simulink model "BLDC_motor_control_v1"  (R2017b)
settings: Solver=FixedStepDiscrete  StartTime=0.0  StopTime=10  FixedStep=1e-5  RelTol=1e-3
values from neighbouring files (symbols this model uses):
  p = 2    [BLDC_model_init.m]
libraries: nesl_utility x41, fl_lib x33, pe_lib x30, simulink x6, pePwmGenerator x2
(part 1 of 2)
settings Model: SimulationMode=accelerator  Creator=proso  LastModifiedBy=proso

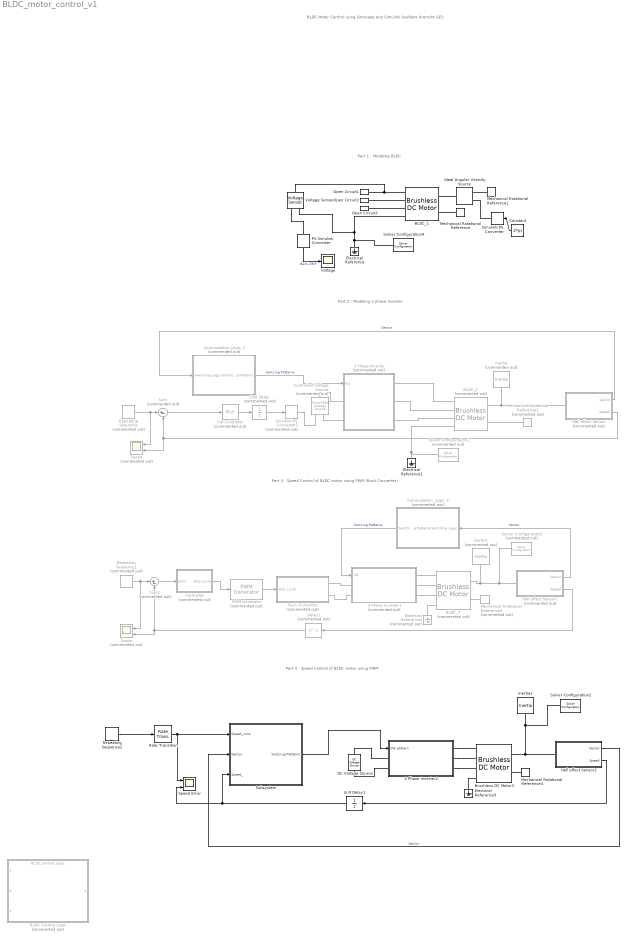
== system BLDC_motor_control_v1 ==
  note: BLDC Motor Control using Simscape and Simulink
      |
      | Soufiane Kremcht GE2
  note: Part 1 : Modeling BLDC
  note: Part 2 : Modeling 3 phase Inverter
  note: Part 3 : Speed Control of BLDC motor using PWM
      | (Buck Converter)
  note: Part 4 : Speed Control of BLDC motor using PWM
  3 Phase Inverter : Subsystem  Commented=on
  3 Phase Inverter1 : Subsystem  Commented=on
  3 Phase Inverter2 : Subsystem
  BLDC Control Logic : ModelReference  Commented=on  ModelNameDialog=BLDC_Control_Logic  SimulationMode=Normal  ModelReferenceVersion=1.23
  BLDC_1 : pe_lib/Machines/Permanent Magnet Rotor/Brushless DC Motor  rotor_param=1  pm_flux_linkage=1 Wb  theta_constant=120 deg  emf_max=9.6 V  DphiDtheta_tab=[0, -.1528, -.1528, .1528, .1528, 0] Wb/rad  back_emf_tab=[0, -9.6, -9.6, 9.6, 9.6, 0] V  rotor_angle_tab=[0, 7.5, 22.5, 37.5, 52.5, 60] deg  w_meas=600 rpm  nPolePairs=1  stator_param=1  Ld=8.5e-3 H  Lq=8.5e-3 H  L0=0 H  Ls=0.0002 H  Lm=0 H  Ms=0.00002 H  Rs=0.04 Ohm  initial_currents=[0, 0, 0] A  axes_param=2  angular_position0=0 deg
      settings: SourceProductName=Simscape Power Systems  SourceProductBaseCode=PS
  BLDC_2 : pe_lib/Machines/Permanent Magnet Rotor/Brushless DC Motor  Commented=on  rotor_param=1  pm_flux_linkage=1 Wb  theta_constant=60 deg  emf_max=9.6 V  DphiDtheta_tab=[0, -.1528, -.1528, .1528, .1528, 0] Wb/rad  back_emf_tab=[0, -9.6, -9.6, 9.6, 9.6, 0] V  rotor_angle_tab=[0, 7.5, 22.5, 37.5, 52.5, 60] deg  w_meas=600 rpm  nPolePairs=2  stator_param=1  Ld=8.5e-3 H  Lq=8.5e-3 H  L0=0 H  Ls=0.0002 H  Lm=0 H  Ms=0.00002 H  Rs=0.04 Ohm  initial_currents=[0, 0, 0] A  axes_param=2  angular_position0=0 deg
      settings: SourceProductName=Simscape Power Systems  SourceProductBaseCode=PS
  "BLDC_3 " : pe_lib/Machines/Permanent Magnet Rotor/Brushless DC Motor  Commented=on  rotor_param=1  pm_flux_linkage=1 Wb  theta_constant=120 deg  emf_max=9.6 V  DphiDtheta_tab=[0, -.1528, -.1528, .1528, .1528, 0] Wb/rad  back_emf_tab=[0, -9.6, -9.6, 9.6, 9.6, 0] V  rotor_angle_tab=[0, 7.5, 22.5, 37.5, 52.5, 60] deg  w_meas=600 rpm  nPolePairs=1  stator_param=1  Ld=8.5e-3 H  Lq=8.5e-3 H  L0=0 H  Ls=0.0002 H  Lm=0 H  Ms=0.00002 H  Rs=0.04 Ohm  initial_currents=[0, 0, 0] A  axes_param=2  angular_position0=0 deg
      settings: SourceProductName=Simscape Power Systems  SourceProductBaseCode=PS
  Brushless DC Motor3 : pe_lib/Machines/Permanent Magnet Rotor/Brushless DC Motor  rotor_param=1  pm_flux_linkage=1 Wb  theta_constant=120 deg  emf_max=9.6 V  DphiDtheta_tab=[0, -.1528, -.1528, .1528, .1528, 0] Wb/rad  back_emf_tab=[0, -9.6, -9.6, 9.6, 9.6, 0] V  rotor_angle_tab=[0, 7.5, 22.5, 37.5, 52.5, 60] deg  w_meas=600 rpm  nPolePairs=1  stator_param=1  Ld=8.5e-3 H  Lq=8.5e-3 H  L0=0 H  Ls=0.0002 H  Lm=0 H  Ms=0.00002 H  Rs=0.04 Ohm  initial_currents=[0, 0, 0] A  axes_param=2  angular_position0=0 deg
      settings: SourceProductName=Simscape Power Systems  SourceProductBaseCode=PS
  Buck Convertor : Subsystem  Commented=on
  Commutation_Logic_2 : Subsystem  Commented=on
  Commutation_Logic_3 : Subsystem  Commented=on
  Constant : Constant  Value=2*pi
  Controlled Voltage Source : fl_lib/Electrical/Electrical Sources/Controlled Voltage Source  Commented=on
  Controller : Subsystem  Commented=on
  DC Voltage Source : fl_lib/Electrical/Electrical Sources/DC Voltage Source  v0=100 V
  Delay1 : Delay  Commented=on  DelayLength=1
  Electrical Reference : fl_lib/Electrical/Electrical Elements/Electrical Reference
  Electrical Reference1 : fl_lib/Electrical/Electrical Elements/Electrical Reference
  Electrical Reference2 : fl_lib/Electrical/Electrical Elements/Electrical Reference  Commented=on
  Electrical Reference3 : fl_lib/Electrical/Electrical Elements/Electrical Reference
  Hall effect Sensor : Subsystem  Commented=on
  Hall effect Sensor1 : Subsystem  Commented=on
  Hall effect Sensor2 : Subsystem
  Ideal Angular Velocity Source : fl_lib/Mechanical/Mechanical Sources/Ideal Angular Velocity Source
  Inertia : fl_lib/Mechanical/Rotational Elements/Inertia  Commented=on  inertia=0.2 kg*m^2  w_specify=off  w_priority=High  w=0 rad/s  w_nominal_specify=off  w_nominal_unit=rad/s  w_nominal_value=1  t_specify=off  t_priority=None  t=0 N*m  t_nominal_specify=off  t_nominal_unit=N*m  t_nominal_value=1
  Inertia1 : fl_lib/Mechanical/Rotational Elements/Inertia  Commented=on  inertia=0.01 kg*m^2  w_specify=off  w_priority=High  w=0 rad/s  w_nominal_specify=off  w_nominal_unit=rad/s  w_nominal_value=1  t_specify=off  t_priority=None  t=0 N*m  t_nominal_specify=off  t_nominal_unit=N*m  t_nominal_value=1
  Inertia2 : fl_lib/Mechanical/Rotational Elements/Inertia  inertia=0.01 kg*m^2  w_specify=off  w_priority=High  w=0 rad/s  w_nominal_specify=off  w_nominal_unit=rad/s  w_nominal_value=1  t_specify=off  t_priority=None  t=0 N*m  t_nominal_specify=off  t_nominal_unit=N*m  t_nominal_value=1
  Mechanical Rotational Reference : fl_lib/Mechanical/Rotational Elements/Mechanical Rotational Reference
  Mechanical Rotational Reference1 : fl_lib/Mechanical/Rotational Elements/Mechanical Rotational Reference
  Mechanical Rotational Reference2 : fl_lib/Mechanical/Rotational Elements/Mechanical Rotational Reference  Commented=on
  Mechanical Rotational Reference3 : fl_lib/Mechanical/Rotational Elements/Mechanical Rotational Reference  Commented=on
  Mechanical Rotational Reference4 : fl_lib/Mechanical/Rotational Elements/Mechanical Rotational Reference
  Open Circuit1 : fl_lib/Electrical/Electrical Elements/Open Circuit  v_specify=off  v_priority=None  v=0 V  v_nominal_specify=off  v_nominal_unit=V  v_nominal_value=1
      settings: SourceProductName=Simscape  SourceProductBaseCode=SS
  Open Circuit2 : fl_lib/Electrical/Electrical Elements/Open Circuit  v_specify=off  v_priority=None  v=0 V  v_nominal_specify=off  v_nominal_unit=V  v_nominal_value=1
      settings: SourceProductName=Simscape  SourceProductBaseCode=SS
  Open Circuit3 : fl_lib/Electrical/Electrical Elements/Open Circuit  v_specify=off  v_priority=None  v=0 V  v_nominal_specify=off  v_nominal_unit=V  v_nominal_value=1
      settings: SourceProductName=Simscape  SourceProductBaseCode=SS
  PID Controller : simulink/Continuous/PID Controller  Commented=on  Controller=PI  TimeDomain=Discrete-time  SampleTime=-1  IntegratorMethod=Forward Euler  FilterMethod=Forward Euler  Form=Parallel  UseFilter=on  ControllerParametersSource=internal  P=0.02  I=5  D=0  N=100  InitialConditionSource=internal  InitialConditionForIntegrator=0  InitialConditionForFilter=0  ExternalReset=none  LimitOutput=off  UpperSaturationLimit=inf  LowerSaturationLimit=-inf  LinearizeAsGain=on  AntiWindupMode=none  Kb=1  TrackingMode=off  Kt=1  PParamMin=[]  PParamMax=[]  IParamMin=[]  IParamMax=[]  DParamMin=[]  DParamMax=[]  NParamMin=[]  NParamMax=[]  KbParamMin=[]  KbParamMax=[]  KtParamMin=[]  KtParamMax=[]  POutMin=[]  POutMax=[]  IOutMin=[]  IOutMax=[]  DOutMin=[]  DOutMax=[]  NOutMin=[]  NOutMax=[]  KbOutMin=[]  KbOutMax=[]  KtOutMin=[]  KtOutMax=[]  IntegratorOutMin=[]  IntegratorOutMax=[]  FilterOutMin=[]  FilterOutMax=[]  SumOutMin=[]  SumOutMax=[]  SumI1OutMin=[]  SumI1OutMax=[]  SumI2OutMin=[]  SumI2OutMax=[]  SumI3OutMin=[]  SumI3OutMax=[]  SumDOutMin=[]  SumDOutMax=[]  SaturationOutMin=[]  SaturationOutMax=[]  IntegratorContinuousStateAttributes=''  IntegratorStateMustResolveToSignalObject=off  IntegratorRTWStateStorageClass=Auto  FilterContinuousStateAttributes=''  FilterStateMustResolveToSignalObject=off  FilterRTWStateStorageClass=Auto  DifferentiatorICPrevScaledInput=0  DifferentiatorOutMin=[]  DifferentiatorOutMax=[]  InitialConditionSetting=State (most efficient)  FilterDiffOutCoefMin=[]  FilterDiffOutCoefMax=[]  SumDenOutMin=[]  SumDenOutMax=[]  SumNumOutMin=[]  SumNumOutMax=[]  ReciprocalOutMin=[]  ReciprocalOutMax=[]  DivideOutMin=[]  DivideOutMax=[]  TunerSelectOption=Transfer Function Based (PID Tuner App)
  PS-Simulink Converter : nesl_utility/PS-Simulink Converter  PhysicalDomain=network_engine_domain  SubClassName=ps_output  LeftPortType=input  RightPortType=output  PseudoPeriodic=off  Frequencies=[]  Unit=1  AffineConversion=off
  PWM Generator : pePwmGenerator/PWM Generator  Commented=on  CarrCount=Up  Tper=0.001  Ts=5e-5
  Rate Transition : RateTransition  OutPortSampleTimeOpt=Inherit  OutPortSampleTime=1e-5
  Repeating Sequence : simulink/Sources/Repeating Sequence  Commented=on  rep_seq_t=[0 0.1 0.2 0.4 0.7 1 1.3 1.7 2]  rep_seq_y=[0 100 100 300 300 600 600 900 900]
  Repeating Sequence1 : simulink/Sources/Repeating Sequence  Commented=on  rep_seq_t=[0 2 2.01 4 4.01 10]  rep_seq_y="[0 20 40  60 80 100]"
  Repeating Sequence2 : simulink/Sources/Repeating Sequence  rep_seq_t=[0 2 3 6 8 10]  rep_seq_y=[0 20 40 50 50 100]
  Scope : Scope  Commented=on  NumInputPorts=2
  Simulink-PS Converter : nesl_utility/Simulink-PS Converter  PhysicalDomain=network_engine_domain  SubClassName=ps_input  LeftPortType=input  RightPortType=output  PseudoPeriodic=off  Frequencies=[]  NoiseDistribution=none  NoiseParameters=[]  Unit=1  AffineConversion=off  FilteringAndDerivatives=provide  SimscapeFilterOrder=1  InputFilterTimeConstant=0.001  UdotUserProvided=0
  Simulink-PS Converter1 : nesl_utility/Simulink-PS Converter  Commented=on  PhysicalDomain=network_engine_domain  SubClassName=ps_input  LeftPortType=input  RightPortType=output  PseudoPeriodic=off  Frequencies=[]  NoiseDistribution=none  NoiseParameters=[]  Unit=1  AffineConversion=off  FilteringAndDerivatives=provide  SimscapeFilterOrder=1  InputFilterTimeConstant=0.001  UdotUserProvided=0
  Solver Configuration1 : nesl_utility/Solver Configuration  Commented=on  PhysicalDomain=network_engine_domain  SubClassName=solver  LeftPortType=input  RightPortType=generic  Accelerate=off  Tones=[]  Harmonics=[]  SimulateNoise=off  Profile=off  UseLocalSampling=off  EnableSwitchedLinearOptims=on  FrequencyDomain=off  UseCCode=off  RelTol=0.001  AbsTol=1e-06  MinStep=1e-09  ToWorkspace=off  RevertToSquareIcSolve=off  NumHomotopyIterations=100  PhasorMode=off  PhasorModeNumHarmonics=1  DoDC=off  ResidualTolerance=1e-09  UseLocalSolver=on  LocalSolverChoice=NE_BACKWARD_EULER_ADVANCER  LocalSolverSampleTime=2e-5  DoFixedCost=on  MaxNonlinIter=4  MaxModeIter=2  LinearAlgebra=Sparse  DelaysMemoryBudget=1024  AutomaticFiltering=off  FilteringTimeConstant=0.001
  Solver Configuration2 : nesl_utility/Solver Configuration  PhysicalDomain=network_engine_domain  SubClassName=solver  LeftPortType=input  RightPortType=generic  Accelerate=off  Tones=[]  Harmonics=[]  SimulateNoise=off  Profile=off  UseLocalSampling=off  EnableSwitchedLinearOptims=on  FrequencyDomain=off  UseCCode=off  RelTol=0.001  AbsTol=1e-06  MinStep=1e-09  ToWorkspace=off  RevertToSquareIcSolve=off  NumHomotopyIterations=100  PhasorMode=off  PhasorModeNumHarmonics=1  DoDC=off  ResidualTolerance=1e-09  UseLocalSolver=on  LocalSolverChoice=NE_BACKWARD_EULER_ADVANCER  LocalSolverSampleTime=1e-5  DoFixedCost=on  MaxNonlinIter=4  MaxModeIter=2  LinearAlgebra=Sparse  DelaysMemoryBudget=1024  AutomaticFiltering=off  FilteringTimeConstant=0.001
  Solver Configuration4 : nesl_utility/Solver Configuration  PhysicalDomain=network_engine_domain  SubClassName=solver  LeftPortType=input  RightPortType=generic  Accelerate=off  Tones=[]  Harmonics=[]  SimulateNoise=off  Profile=off  UseLocalSampling=off  EnableSwitchedLinearOptims=on  FrequencyDomain=off  UseCCode=off  RelTol=0.001  AbsTol=1e-06  MinStep=1e-09  ToWorkspace=off  RevertToSquareIcSolve=off  NumHomotopyIterations=100  PhasorMode=off  PhasorModeNumHarmonics=1  DoDC=off  ResidualTolerance=1e-09  UseLocalSolver=on  LocalSolverChoice=NE_BACKWARD_EULER_ADVANCER  LocalSolverSampleTime=0.001  DoFixedCost=on  MaxNonlinIter=3  MaxModeIter=2  LinearAlgebra=Sparse  DelaysMemoryBudget=1024  AutomaticFiltering=off  FilteringTimeConstant=0.001
  Solver Configuration5 : nesl_utility/Solver Configuration  Commented=on  PhysicalDomain=network_engine_domain  SubClassName=solver  LeftPortType=input  RightPortType=generic  Accelerate=off  Tones=[]  Harmonics=[]  SimulateNoise=off  Profile=off  UseLocalSampling=off  EnableSwitchedLinearOptims=on  FrequencyDomain=off  UseCCode=off  RelTol=0.001  AbsTol=1e-06  MinStep=1e-09  ToWorkspace=off  RevertToSquareIcSolve=off  NumHomotopyIterations=100  PhasorMode=off  PhasorModeNumHarmonics=1  DoDC=off  ResidualTolerance=1e-09  UseLocalSolver=on  LocalSolverChoice=NE_BACKWARD_EULER_ADVANCER  LocalSolverSampleTime=1e-5  DoFixedCost=on  MaxNonlinIter=4  MaxModeIter=2  LinearAlgebra=Sparse  DelaysMemoryBudget=1024  AutomaticFiltering=off  FilteringTimeConstant=0.001
  "Speed " : Scope  Commented=on  NumInputPorts=2
  Speed Error : Scope  NumInputPorts=2
  Subsystem : Subsystem
  Sum : Sum  Commented=on  Inputs=|+-
  Sum1 : Sum  Commented=on  Inputs=|+-
  Unit Delay : UnitDelay  Commented=on  SampleTime=-1
  Unit Delay1 : UnitDelay  SampleTime=-1
  "Voltage " : Scope
  Voltage Sensor : fl_lib/Electrical/Electrical Sensors/Voltage Sensor
  wires:
  PS-Simulink Converter/1 -> "Voltage "/1  "Back-EMF"
  Constant/1 -> Simulink-PS Converter/1
  Hall effect Sensor/1(Sector) -> Commutation_Logic_2/1(Switching Logic)  "Sector"
  Commutation_Logic_2/1(Switching Patterns) -> 3 Phase Inverter/1(In1)  "Switcing Patterns"
  Hall effect Sensor/2(Speed) -> "Speed "/2, Sum/2
  Repeating Sequence/1 -> "Speed "/1, Sum/1
  Sum/1 -> PID Controller/1
  PID Controller/1 -> Unit Delay/1
  Commutation_Logic_3/1(Switching Patterns) -> 3 Phase Inverter1/1(In1)  "Switcing Patterns"
  Hall effect Sensor1/2(Speed) -> Delay1/1
  Repeating Sequence1/1 -> Scope/1, Sum1/1
  Hall effect Sensor1/1(Sector) -> Commutation_Logic_3/1(Switching Logic)  "Sector"
  Sum1/1 -> Controller/1(error)
  Controller/1(duty cycle) -> PWM Generator/1
  PWM Generator/1 -> Buck Convertor/1(duty cycle)
  Delay1/1 -> Scope/2, Sum1/2
  Hall effect Sensor2/2(Speed) -> Unit Delay1/1
  Unit Delay/1 -> Simulink-PS Converter1/1
  Repeating Sequence2/1 -> Rate Transition/1
  Hall effect Sensor2/1(Sector) -> Subsystem/2(Sector)  "Sector"
  Subsystem/1(Switcing Patterns) -> 3 Phase Inverter2/1(SW pattern)
  Unit Delay1/1 -> Subsystem/3(Speed_), Speed Error/2
  Rate Transition/1 -> Subsystem/1(Speed_cmd), Speed Error/1
  connections:
  Open Circuit1/LConn1 -- Voltage Sensor/LConn1 -- BLDC_1/LConn1
  Open Circuit2/LConn1 -- BLDC_1/LConn2
  Open Circuit3/LConn1 -- BLDC_1/LConn3
  BLDC_1/LConn4 -- Voltage Sensor/RConn2 -- Solver Configuration4/RConn1 -- Electrical Reference/LConn1
  Ideal Angular Velocity Source/LConn1 -- BLDC_1/RConn1
  Simulink-PS Converter/RConn1 -- Ideal Angular Velocity Source/RConn1
  Mechanical Rotational Reference/LConn1 -- BLDC_1/RConn2
  Mechanical Rotational Reference1/LConn1 -- Ideal Angular Velocity Source/RConn2
  Voltage Sensor/RConn1 -- PS-Simulink Converter/LConn1
  Mechanical Rotational Reference2/LConn1 -- BLDC_2/RConn2
  BLDC_2/LConn4 -- Solver Configuration1/RConn1 -- Electrical Reference1/LConn1
  BLDC_2/RConn1 -- Hall effect Sensor/LConn1 -- Inertia/LConn1
  3 Phase Inverter/RConn1 -- BLDC_2/LConn1
  3 Phase Inverter/RConn2 -- BLDC_2/LConn2
  3 Phase Inverter/RConn3 -- BLDC_2/LConn3
  Controlled Voltage Source/LConn1 -- 3 Phase Inverter/LConn1
  Controlled Voltage Source/RConn2 -- 3 Phase Inverter/LConn2
  "BLDC_3 "/RConn1 -- Inertia1/LConn1 -- Solver Configuration5/RConn1 -- Hall effect Sensor1/LConn1
  Mechanical Rotational Reference3/LConn1 -- "BLDC_3 "/RConn2
  3 Phase Inverter1/RConn3 -- "BLDC_3 "/LConn3
  3 Phase Inverter1/RConn1 -- "BLDC_3 "/LConn1
  3 Phase Inverter1/RConn2 -- "BLDC_3 "/LConn2
  "BLDC_3 "/LConn4 -- Electrical Reference2/LConn1
  3 Phase Inverter1/LConn1 -- Buck Convertor/RConn1
  3 Phase Inverter1/LConn2 -- Buck Convertor/RConn2
  Mechanical Rotational Reference4/LConn1 -- Brushless DC Motor3/RConn2
  Brushless DC Motor3/LConn4 -- Electrical Reference3/LConn1
  DC Voltage Source/RConn1 -- 3 Phase Inverter2/LConn2
  3 Phase Inverter2/RConn2 -- Brushless DC Motor3/LConn2
  3 Phase Inverter2/RConn3 -- Brushless DC Motor3/LConn3
  3 Phase Inverter2/RConn1 -- Brushless DC Motor3/LConn1
  DC Voltage Source/LConn1 -- 3 Phase Inverter2/LConn1
  Simulink-PS Converter1/RConn1 -- Controlled Voltage Source/RConn1
  Brushless DC Motor3/RConn1 -- Hall effect Sensor2/LConn1 -- Solver Configuration2/RConn1 -- Inertia2/LConn1

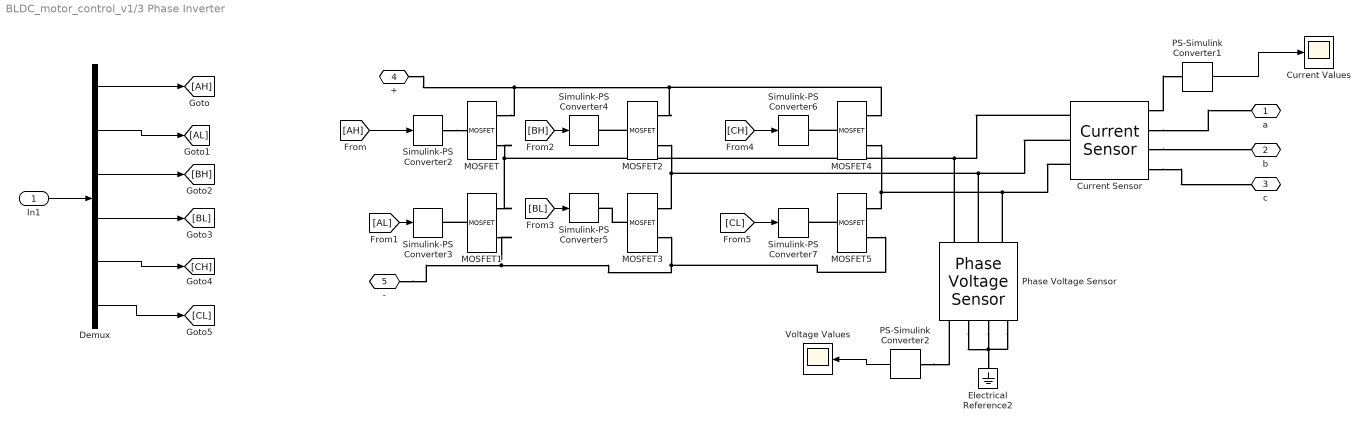
== system BLDC_motor_control_v1/3 Phase Inverter ==
  In1 : Inport
  Current Sensor : pe_lib/Sensors/Current Sensor
      settings: SourceProductName=Simscape Power Systems  SourceProductBaseCode=PS
  Current Values : Scope
  Demux : Demux  Outputs=6
  Electrical Reference2 : fl_lib/Electrical/Electrical Elements/Electrical Reference
  MOSFET{,1..5} (6 alike) : pe_lib/Semiconductors/Fundamental Components/MOSFET  Rds=0.01 Ohm  Goff=1e-6 1/Ohm  Vth=0.5 V  diode_param=2  diode_Vf=0.1 V  diode_Ron=0.001 Ohm  diode_Goff=1e-5 1/Ohm  diode_C=5e-8 F  diode_iRM=-235 A  diode_iF=300 A  diode_idot=-50 A/us  diode_trr_param=1  diode_trr_factor=3  diode_trr=15 us  diode_Qrr=1.5e+3 s*uA  thermal_loss_option=2  Voff=300 V  Tau=1e-4 s  Tj=[ 298.15 398.15 ] K  Iout_scalar=600 A  Eon_scalar=0.02286 J  Eoff_scalar=0.01714 J  Von_scalar=2.7 V  Iout_data=[ 0 10 50 100 200 400 600 ] A  Eon_data=[ 0 2.9e-4 0.00143 0.00286 0.00571 0.01314 0.02286; 0 5.7e-4 0.00263 0.00514 0.01029 0.02057 0.03029 ] J  Eoff_data=[ 0 2.1e-4 0.00107 0.00214 0.00429 0.009859999999999999 0.01714; 0 4.3e-4 0.00197 0.00386 0.00771 0.01543 0.02271 ] J  Von_data=[ 0 1.1 1.3 1.45 1.75 2.25 2.7; 0 1 1.15 1.35 1.7 2.35 3 ] V
      settings: SourceProductName=Simscape Power Systems  SourceProductBaseCode=PS
  PS-Simulink Converter1 : nesl_utility/PS-Simulink Converter  PhysicalDomain=network_engine_domain  SubClassName=ps_output  LeftPortType=input  RightPortType=output  PseudoPeriodic=off  Frequencies=[]  Unit=1  AffineConversion=off
  PS-Simulink Converter2 : nesl_utility/PS-Simulink Converter  PhysicalDomain=network_engine_domain  SubClassName=ps_output  LeftPortType=input  RightPortType=output  PseudoPeriodic=off  Frequencies=[]  Unit=1  AffineConversion=off
  Phase Voltage Sensor : pe_lib/Sensors/Phase Voltage Sensor
      settings: SourceProductName=Simscape Power Systems  SourceProductBaseCode=PS
  Simulink-PS Converter{2..7} (6 alike) : nesl_utility/Simulink-PS Converter  PhysicalDomain=network_engine_domain  SubClassName=ps_input  LeftPortType=input  RightPortType=output  PseudoPeriodic=off  Frequencies=[]  NoiseDistribution=none  NoiseParameters=[]  Unit=1  AffineConversion=off  FilteringAndDerivatives=provide  SimscapeFilterOrder=1  InputFilterTimeConstant=0.001  UdotUserProvided=0
  Voltage Values : Scope
  a : PMIOPort  Port=1  Side=Right
  b : PMIOPort  Port=2  Side=Right
  c : PMIOPort  Port=3  Side=Right
  + : PMIOPort  Port=4  Side=Left
  - : PMIOPort  Port=5  Side=Left
  wires:
  Demux/4 -> [BL]
  [CH] -> Simulink-PS Converter6/1
  Demux/3 -> [BH]
  In1/1 -> Demux/1
  [AH] -> Simulink-PS Converter2/1
  Demux/1 -> [AH]
  PS-Simulink Converter2/1 -> Voltage Values/1
  Demux/5 -> [CH]
  Demux/6 -> [CL]
  [CL] -> Simulink-PS Converter7/1
  [BL] -> Simulink-PS Converter5/1
  [BH] -> Simulink-PS Converter4/1
  PS-Simulink Converter1/1 -> Current Values/1
  [AL] -> Simulink-PS Converter3/1
  Demux/2 -> [AL]
  connections:
  +/RConn1 -- MOSFET/RConn1 -- MOSFET4/RConn1 -- MOSFET2/RConn1
  Phase Voltage Sensor/LConn2 -- Current Sensor/LConn2 -- MOSFET3/RConn1 -- MOSFET2/RConn2
  MOSFET4/LConn1 -- Simulink-PS Converter6/RConn1
  MOSFET/RConn2 -- MOSFET1/RConn1 -- Phase Voltage Sensor/LConn1 -- Current Sensor/LConn1
  Phase Voltage Sensor/LConn3 -- Current Sensor/LConn3 -- MOSFET5/RConn1 -- MOSFET4/RConn2
  MOSFET1/RConn2 -- -/RConn1 -- MOSFET5/RConn2 -- MOSFET3/RConn2
  PS-Simulink Converter2/LConn1 -- Phase Voltage Sensor/RConn1
  Current Sensor/RConn2 -- a/RConn1
  Simulink-PS Converter2/RConn1 -- MOSFET/LConn1
  MOSFET5/LConn1 -- Simulink-PS Converter7/RConn1
  Current Sensor/RConn3 -- b/RConn1
  Current Sensor/RConn1 -- PS-Simulink Converter1/LConn1
  MOSFET3/LConn1 -- Simulink-PS Converter5/RConn1
  MOSFET2/LConn1 -- Simulink-PS Converter4/RConn1
  MOSFET1/LConn1 -- Simulink-PS Converter3/RConn1
  Phase Voltage Sensor/RConn2 -- Phase Voltage Sensor/RConn4 -- Phase Voltage Sensor/RConn3 -- Electrical Reference2/LConn1
  Current Sensor/RConn4 -- c/RConn1

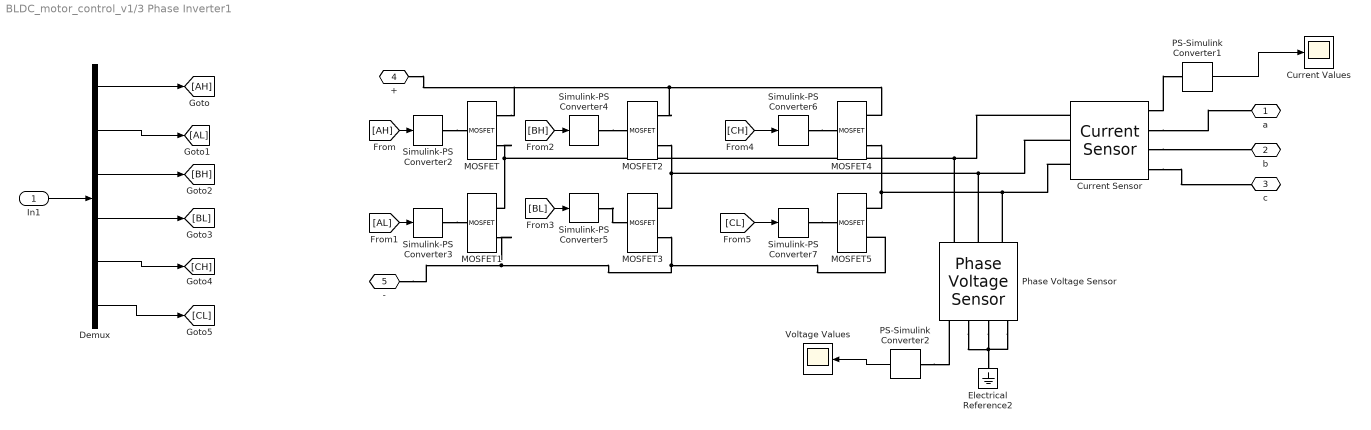
== system BLDC_motor_control_v1/3 Phase Inverter1 ==
  In1 : Inport
  Current Sensor : pe_lib/Sensors/Current Sensor
      settings: SourceProductName=Simscape Power Systems  SourceProductBaseCode=PS
  Current Values : Scope
  Demux : Demux  Outputs=6
  Electrical Reference2 : fl_lib/Electrical/Electrical Elements/Electrical Reference
  MOSFET{,1..5} (6 alike) : pe_lib/Semiconductors/Fundamental Components/MOSFET  Rds=0.01 Ohm  Goff=1e-6 1/Ohm  Vth=2 V  diode_param=2  diode_Vf=0.8 V  diode_Ron=0.001 Ohm  diode_Goff=1e-5 1/Ohm  diode_C=5e-8 F  diode_iRM=-235 A  diode_iF=300 A  diode_idot=-50 A/us  diode_trr_param=1  diode_trr_factor=3  diode_trr=15 us  diode_Qrr=1.5e+3 s*uA  thermal_loss_option=2  Voff=300 V  Tau=1e-4 s  Tj=[ 298.15 398.15 ] K  Iout_scalar=600 A  Eon_scalar=0.02286 J  Eoff_scalar=0.01714 J  Von_scalar=2.7 V  Iout_data=[ 0 10 50 100 200 400 600 ] A  Eon_data=[ 0 2.9e-4 0.00143 0.00286 0.00571 0.01314 0.02286; 0 5.7e-4 0.00263 0.00514 0.01029 0.02057 0.03029 ] J  Eoff_data=[ 0 2.1e-4 0.00107 0.00214 0.00429 0.009859999999999999 0.01714; 0 4.3e-4 0.00197 0.00386 0.00771 0.01543 0.02271 ] J  Von_data=[ 0 1.1 1.3 1.45 1.75 2.25 2.7; 0 1 1.15 1.35 1.7 2.35 3 ] V
      settings: SourceProductName=Simscape Power Systems  SourceProductBaseCode=PS
  PS-Simulink Converter1 : nesl_utility/PS-Simulink Converter  PhysicalDomain=network_engine_domain  SubClassName=ps_output  LeftPortType=input  RightPortType=output  PseudoPeriodic=off  Frequencies=[]  Unit=1  AffineConversion=off
  PS-Simulink Converter2 : nesl_utility/PS-Simulink Converter  PhysicalDomain=network_engine_domain  SubClassName=ps_output  LeftPortType=input  RightPortType=output  PseudoPeriodic=off  Frequencies=[]  Unit=1  AffineConversion=off
  Phase Voltage Sensor : pe_lib/Sensors/Phase Voltage Sensor
      settings: SourceProductName=Simscape Power Systems  SourceProductBaseCode=PS
  Simulink-PS Converter{2..7} (6 alike) : nesl_utility/Simulink-PS Converter  PhysicalDomain=network_engine_domain  SubClassName=ps_input  LeftPortType=input  RightPortType=output  PseudoPeriodic=off  Frequencies=[]  NoiseDistribution=none  NoiseParameters=[]  Unit=1  AffineConversion=off  FilteringAndDerivatives=provide  SimscapeFilterOrder=1  InputFilterTimeConstant=0.001  UdotUserProvided=0
  Voltage Values : Scope
  a : PMIOPort  Port=1  Side=Right
  b : PMIOPort  Port=2  Side=Right
  c : PMIOPort  Port=3  Side=Right
  + : PMIOPort  Port=4  Side=Left
  - : PMIOPort  Port=5  Side=Left
  wires:
  Demux/4 -> [BL]
  [CH] -> Simulink-PS Converter6/1
  Demux/3 -> [BH]
  In1/1 -> Demux/1
  [AH] -> Simulink-PS Converter2/1
  Demux/1 -> [AH]
  PS-Simulink Converter2/1 -> Voltage Values/1
  Demux/5 -> [CH]
  Demux/6 -> [CL]
  [CL] -> Simulink-PS Converter7/1
  [BL] -> Simulink-PS Converter5/1
  [BH] -> Simulink-PS Converter4/1
  PS-Simulink Converter1/1 -> Current Values/1
  [AL] -> Simulink-PS Converter3/1
  Demux/2 -> [AL]
  connections:
  MOSFET2/RConn1 -- MOSFET4/RConn1 -- MOSFET/RConn1 -- +/RConn1
  Current Sensor/LConn2 -- MOSFET2/RConn2 -- MOSFET3/RConn1 -- Phase Voltage Sensor/LConn2
  Simulink-PS Converter6/RConn1 -- MOSFET4/LConn1
  Current Sensor/LConn1 -- MOSFET/RConn2 -- MOSFET1/RConn1 -- Phase Voltage Sensor/LConn1
  Current Sensor/LConn3 -- MOSFET4/RConn2 -- MOSFET5/RConn1 -- Phase Voltage Sensor/LConn3
  MOSFET1/RConn2 -- MOSFET3/RConn2 -- MOSFET5/RConn2 -- -/RConn1
  PS-Simulink Converter2/LConn1 -- Phase Voltage Sensor/RConn1
  Current Sensor/RConn2 -- a/RConn1
  Simulink-PS Converter2/RConn1 -- MOSFET/LConn1
  Simulink-PS Converter7/RConn1 -- MOSFET5/LConn1
  Current Sensor/RConn3 -- b/RConn1
  Current Sensor/RConn1 -- PS-Simulink Converter1/LConn1
  Simulink-PS Converter5/RConn1 -- MOSFET3/LConn1
  Simulink-PS Converter4/RConn1 -- MOSFET2/LConn1
  Simulink-PS Converter3/RConn1 -- MOSFET1/LConn1
  Phase Voltage Sensor/RConn3 -- Phase Voltage Sensor/RConn2 -- Electrical Reference2/LConn1 -- Phase Voltage Sensor/RConn4
  Current Sensor/RConn4 -- c/RConn1

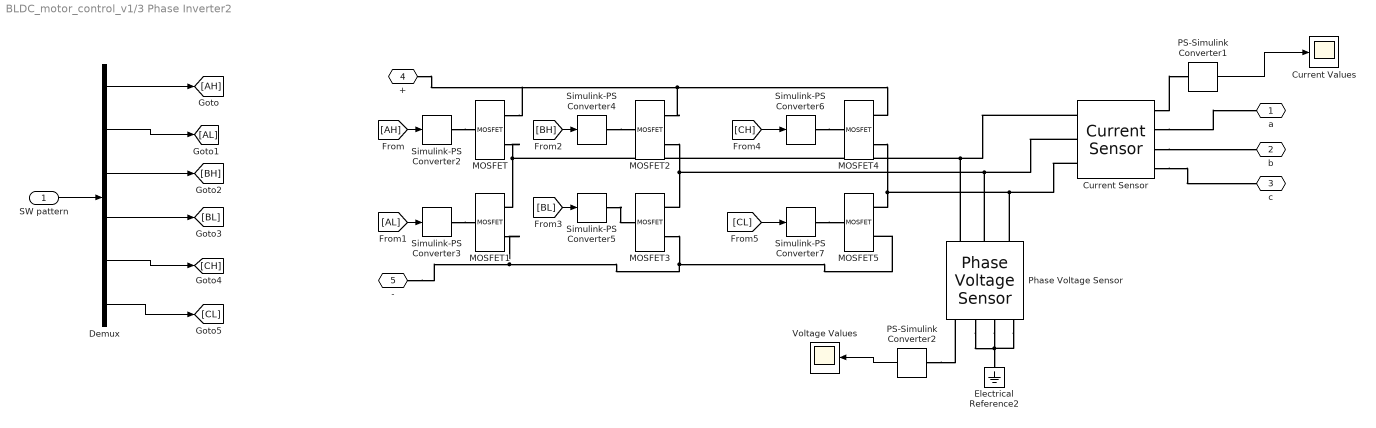
== system BLDC_motor_control_v1/3 Phase Inverter2 ==
  SW pattern : Inport
  Current Sensor : pe_lib/Sensors/Current Sensor
      settings: SourceProductName=Simscape Power Systems  SourceProductBaseCode=PS
  Current Values : Scope
  Demux : Demux  Outputs=6
  Electrical Reference2 : fl_lib/Electrical/Electrical Elements/Electrical Reference
  MOSFET{,1..5} (6 alike) : pe_lib/Semiconductors/Fundamental Components/MOSFET  Rds=0.01 Ohm  Goff=1e-6 1/Ohm  Vth=2 V  diode_param=2  diode_Vf=0.8 V  diode_Ron=0.001 Ohm  diode_Goff=1e-5 1/Ohm  diode_C=5e-8 F  diode_iRM=-235 A  diode_iF=300 A  diode_idot=-50 A/us  diode_trr_param=1  diode_trr_factor=3  diode_trr=15 us  diode_Qrr=1.5e+3 s*uA  thermal_loss_option=2  Voff=300 V  Tau=1e-4 s  Tj=[ 298.15 398.15 ] K  Iout_scalar=600 A  Eon_scalar=0.02286 J  Eoff_scalar=0.01714 J  Von_scalar=2.7 V  Iout_data=[ 0 10 50 100 200 400 600 ] A  Eon_data=[ 0 2.9e-4 0.00143 0.00286 0.00571 0.01314 0.02286; 0 5.7e-4 0.00263 0.00514 0.01029 0.02057 0.03029 ] J  Eoff_data=[ 0 2.1e-4 0.00107 0.00214 0.00429 0.009859999999999999 0.01714; 0 4.3e-4 0.00197 0.00386 0.00771 0.01543 0.02271 ] J  Von_data=[ 0 1.1 1.3 1.45 1.75 2.25 2.7; 0 1 1.15 1.35 1.7 2.35 3 ] V
      settings: SourceProductName=Simscape Power Systems  SourceProductBaseCode=PS
  PS-Simulink Converter1 : nesl_utility/PS-Simulink Converter  PhysicalDomain=network_engine_domain  SubClassName=ps_output  LeftPortType=input  RightPortType=output  PseudoPeriodic=off  Frequencies=[]  Unit=1  AffineConversion=off
  PS-Simulink Converter2 : nesl_utility/PS-Simulink Converter  PhysicalDomain=network_engine_domain  SubClassName=ps_output  LeftPortType=input  RightPortType=output  PseudoPeriodic=off  Frequencies=[]  Unit=1  AffineConversion=off
  Phase Voltage Sensor : pe_lib/Sensors/Phase Voltage Sensor
      settings: SourceProductName=Simscape Power Systems  SourceProductBaseCode=PS
  Simulink-PS Converter{2..7} (6 alike) : nesl_utility/Simulink-PS Converter  PhysicalDomain=network_engine_domain  SubClassName=ps_input  LeftPortType=input  RightPortType=output  PseudoPeriodic=off  Frequencies=[]  NoiseDistribution=none  NoiseParameters=[]  Unit=1  AffineConversion=off  FilteringAndDerivatives=provide  SimscapeFilterOrder=1  InputFilterTimeConstant=0.001  UdotUserProvided=0
  Voltage Values : Scope
  a : PMIOPort  Port=1  Side=Right
  b : PMIOPort  Port=2  Side=Right
  c : PMIOPort  Port=3  Side=Right
  + : PMIOPort  Port=4  Side=Left
  - : PMIOPort  Port=5  Side=Left
  wires:
  Demux/4 -> [BL]
  [CH] -> Simulink-PS Converter6/1
  Demux/3 -> [BH]
  SW pattern/1 -> Demux/1
  [AH] -> Simulink-PS Converter2/1
  Demux/1 -> [AH]
  PS-Simulink Converter2/1 -> Voltage Values/1
  Demux/5 -> [CH]
  Demux/6 -> [CL]
  [CL] -> Simulink-PS Converter7/1
  [BL] -> Simulink-PS Converter5/1
  [BH] -> Simulink-PS Converter4/1
  PS-Simulink Converter1/1 -> Current Values/1
  [AL] -> Simulink-PS Converter3/1
  Demux/2 -> [AL]
  connections:
  MOSFET2/RConn1 -- MOSFET4/RConn1 -- MOSFET/RConn1 -- +/RConn1
  Current Sensor/LConn2 -- MOSFET2/RConn2 -- MOSFET3/RConn1 -- Phase Voltage Sensor/LConn2
  Simulink-PS Converter6/RConn1 -- MOSFET4/LConn1
  Current Sensor/LConn1 -- MOSFET/RConn2 -- MOSFET1/RConn1 -- Phase Voltage Sensor/LConn1
  Current Sensor/LConn3 -- MOSFET4/RConn2 -- MOSFET5/RConn1 -- Phase Voltage Sensor/LConn3
  MOSFET1/RConn2 -- MOSFET3/RConn2 -- MOSFET5/RConn2 -- -/RConn1
  PS-Simulink Converter2/LConn1 -- Phase Voltage Sensor/RConn1
  Current Sensor/RConn2 -- a/RConn1
  Simulink-PS Converter2/RConn1 -- MOSFET/LConn1
  Simulink-PS Converter7/RConn1 -- MOSFET5/LConn1
  Current Sensor/RConn3 -- b/RConn1
  Current Sensor/RConn1 -- PS-Simulink Converter1/LConn1
  Simulink-PS Converter5/RConn1 -- MOSFET3/LConn1
  Simulink-PS Converter4/RConn1 -- MOSFET2/LConn1
  Simulink-PS Converter3/RConn1 -- MOSFET1/LConn1
  Phase Voltage Sensor/RConn3 -- Phase Voltage Sensor/RConn2 -- Electrical Reference2/LConn1 -- Phase Voltage Sensor/RConn4
  Current Sensor/RConn4 -- c/RConn1

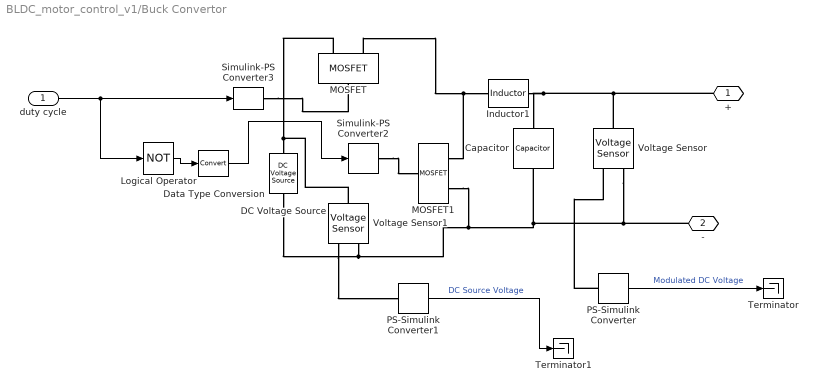
== system BLDC_motor_control_v1/Buck Convertor ==
  duty cycle : Inport
  Capacitor : fl_lib/Electrical/Electrical Elements/Capacitor  c=1e-6 F  r=1e-6 Ohm  g=0 1/Ohm  i_specify=off  i_priority=None  i=0 A  i_nominal_specify=off  i_nominal_unit=A  i_nominal_value=1  v_specify=off  v_priority=None  v=0 V  v_nominal_specify=off  v_nominal_unit=V  v_nominal_value=1  vc_specify=off  vc_priority=High  vc=0 V  vc_nominal_specify=off  vc_nominal_unit=V  vc_nominal_value=1
  DC Voltage Source : fl_lib/Electrical/Electrical Sources/DC Voltage Source  v0=1 V
  Data Type Conversion : DataTypeConversion
  Inductor1 : fl_lib/Electrical/Electrical Elements/Inductor  l=1e-6 H  r=0 Ohm  g=1e-9 1/Ohm  i_specify=off  i_priority=None  i=0 A  i_nominal_specify=off  i_nominal_unit=A  i_nominal_value=1  v_specify=off  v_priority=None  v=0 V  v_nominal_specify=off  v_nominal_unit=V  v_nominal_value=1  i_L_specify=off  i_L_priority=High  i_L=0 A  i_L_nominal_specify=off  i_L_nominal_unit=A  i_L_nominal_value=1
  Logical Operator : Logic  Operator=NOT  AllPortsSameDT=off  OutDataTypeStr=boolean
  MOSFET : pe_lib/Semiconductors/Fundamental Components/MOSFET  Rds=0.0001 Ohm  Goff=1e-6 1/Ohm  Vth=1 V  diode_param=2  diode_Vf=0.1 V  diode_Ron=0.001 Ohm  diode_Goff=1e-5 1/Ohm  diode_C=5e-8 F  diode_iRM=-235 A  diode_iF=300 A  diode_idot=-50 A/us  diode_trr_param=1  diode_trr_factor=3  diode_trr=15 us  diode_Qrr=1.5e+3 s*uA  thermal_loss_option=2  Voff=300 V  Tau=1e-4 s  Tj=[ 298.15 398.15 ] K  Iout_scalar=600 A  Eon_scalar=0.02286 J  Eoff_scalar=0.01714 J  Von_scalar=2.7 V  Iout_data=[ 0 10 50 100 200 400 600 ] A  Eon_data=[ 0 2.9e-4 0.00143 0.00286 0.00571 0.01314 0.02286; 0 5.7e-4 0.00263 0.00514 0.01029 0.02057 0.03029 ] J  Eoff_data=[ 0 2.1e-4 0.00107 0.00214 0.00429 0.009859999999999999 0.01714; 0 4.3e-4 0.00197 0.00386 0.00771 0.01543 0.02271 ] J  Von_data=[ 0 1.1 1.3 1.45 1.75 2.25 2.7; 0 1 1.15 1.35 1.7 2.35 3 ] V
      settings: SourceProductName=Simscape Power Systems  SourceProductBaseCode=PS
  MOSFET1 : pe_lib/Semiconductors/Fundamental Components/MOSFET  Rds=0.0001 Ohm  Goff=1e-6 1/Ohm  Vth=1 V  diode_param=2  diode_Vf=0.1 V  diode_Ron=0.001 Ohm  diode_Goff=1e-5 1/Ohm  diode_C=5e-8 F  diode_iRM=-235 A  diode_iF=300 A  diode_idot=-50 A/us  diode_trr_param=1  diode_trr_factor=3  diode_trr=15 us  diode_Qrr=1.5e+3 s*uA  thermal_loss_option=2  Voff=300 V  Tau=1e-4 s  Tj=[ 298.15 398.15 ] K  Iout_scalar=600 A  Eon_scalar=0.02286 J  Eoff_scalar=0.01714 J  Von_scalar=2.7 V  Iout_data=[ 0 10 50 100 200 400 600 ] A  Eon_data=[ 0 2.9e-4 0.00143 0.00286 0.00571 0.01314 0.02286; 0 5.7e-4 0.00263 0.00514 0.01029 0.02057 0.03029 ] J  Eoff_data=[ 0 2.1e-4 0.00107 0.00214 0.00429 0.009859999999999999 0.01714; 0 4.3e-4 0.00197 0.00386 0.00771 0.01543 0.02271 ] J  Von_data=[ 0 1.1 1.3 1.45 1.75 2.25 2.7; 0 1 1.15 1.35 1.7 2.35 3 ] V
      settings: SourceProductName=Simscape Power Systems  SourceProductBaseCode=PS
  PS-Simulink Converter : nesl_utility/PS-Simulink Converter  PhysicalDomain=network_engine_domain  SubClassName=ps_output  LeftPortType=input  RightPortType=output  PseudoPeriodic=off  Frequencies=[]  Unit=1  AffineConversion=off
  PS-Simulink Converter1 : nesl_utility/PS-Simulink Converter  PhysicalDomain=network_engine_domain  SubClassName=ps_output  LeftPortType=input  RightPortType=output  PseudoPeriodic=off  Frequencies=[]  Unit=1  AffineConversion=off
  Simulink-PS Converter2 : nesl_utility/Simulink-PS Converter  PhysicalDomain=network_engine_domain  SubClassName=ps_input  LeftPortType=input  RightPortType=output  PseudoPeriodic=off  Frequencies=[]  NoiseDistribution=none  NoiseParameters=[]  Unit=1  AffineConversion=off  FilteringAndDerivatives=provide  SimscapeFilterOrder=1  InputFilterTimeConstant=0.001  UdotUserProvided=0
  Simulink-PS Converter3 : nesl_utility/Simulink-PS Converter  PhysicalDomain=network_engine_domain  SubClassName=ps_input  LeftPortType=input  RightPortType=output  PseudoPeriodic=off  Frequencies=[]  NoiseDistribution=none  NoiseParameters=[]  Unit=1  AffineConversion=off  FilteringAndDerivatives=provide  SimscapeFilterOrder=1  InputFilterTimeConstant=0.001  UdotUserProvided=0
  Terminator : Terminator
  Terminator1 : Terminator
  Voltage Sensor : fl_lib/Electrical/Electrical Sensors/Voltage Sensor
  Voltage Sensor1 : fl_lib/Electrical/Electrical Sensors/Voltage Sensor
  + : PMIOPort  Port=1  Side=Right
  - : PMIOPort  Port=2  Side=Right
  wires:
  Data Type Conversion/1 -> Simulink-PS Converter2/1
  Logical Operator/1 -> Data Type Conversion/1
  duty cycle/1 -> Logical Operator/1, Simulink-PS Converter3/1
  PS-Simulink Converter/1 -> Terminator/1  "Modulated DC Voltage"
  PS-Simulink Converter1/1 -> Terminator1/1  "DC Source Voltage"
  connections:
  Inductor1/RConn1 -- Voltage Sensor/LConn1 -- +/RConn1 -- Capacitor/LConn1
  MOSFET/RConn2 -- MOSFET1/RConn1 -- Inductor1/LConn1
  MOSFET1/RConn2 -- DC Voltage Source/RConn1 -- Voltage Sensor1/RConn2 -- Voltage Sensor/RConn2 -- -/RConn1 -- Capacitor/RConn1
  MOSFET/RConn1 -- Voltage Sensor1/LConn1 -- DC Voltage Source/LConn1
  Simulink-PS Converter3/RConn1 -- MOSFET/LConn1
  Simulink-PS Converter2/RConn1 -- MOSFET1/LConn1
  PS-Simulink Converter/LConn1 -- Voltage Sensor/RConn1
  Voltage Sensor1/RConn1 -- PS-Simulink Converter1/LConn1

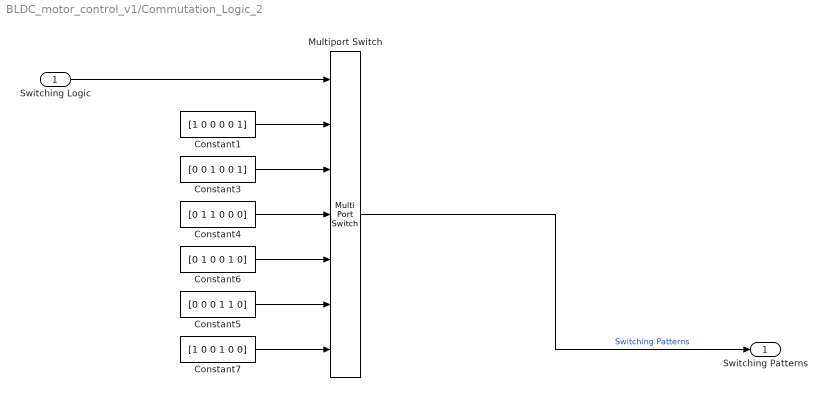
== system BLDC_motor_control_v1/Commutation_Logic_2 ==
  Switching Logic : Inport
  Constant1 : Constant  Value=[1 0 0 0 0 1]
  Constant3 : Constant  Value=[0 0 1 0 0 1]
  Constant4 : Constant  Value=[0 1 1 0 0 0]
  Constant5 : Constant  Value=[0 0 0 1 1 0]
  Constant6 : Constant  Value=[0 1 0 0 1 0]
  Constant7 : Constant  Value=[1 0 0 1 0 0]
  Multiport Switch : MultiPortSwitch  Inputs=6
  Switching Patterns : Outport
  wires:
  Constant4/1 -> Multiport Switch/4
  Constant3/1 -> Multiport Switch/3
  Constant7/1 -> Multiport Switch/7
  Switching Logic/1 -> Multiport Switch/1
  Multiport Switch/1 -> Switching Patterns/1  "Switching Patterns"
  Constant5/1 -> Multiport Switch/6
  Constant6/1 -> Multiport Switch/5
  Constant1/1 -> Multiport Switch/2

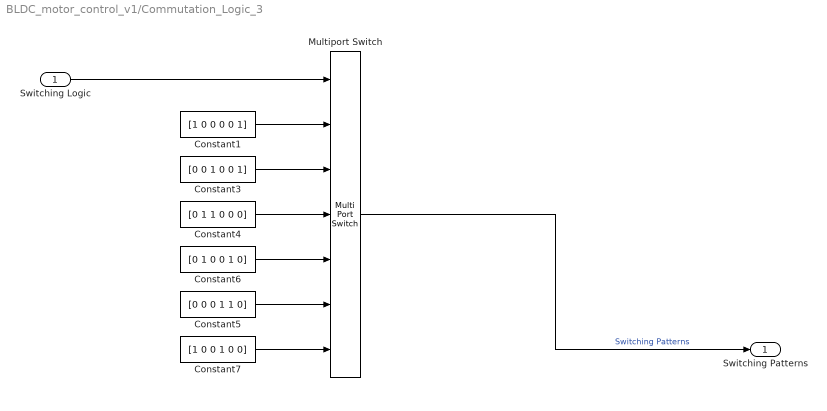
== system BLDC_motor_control_v1/Commutation_Logic_3 ==
  Switching Logic : Inport
  Constant1 : Constant  Value=[1 0 0 0 0 1]
  Constant3 : Constant  Value=[0 0 1 0 0 1]
  Constant4 : Constant  Value=[0 1 1 0 0 0]
  Constant5 : Constant  Value=[0 0 0 1 1 0]
  Constant6 : Constant  Value=[0 1 0 0 1 0]
  Constant7 : Constant  Value=[1 0 0 1 0 0]
  Multiport Switch : MultiPortSwitch  Inputs=6
  Switching Patterns : Outport
  wires:
  Switching Logic/1 -> Multiport Switch/1
  Multiport Switch/1 -> Switching Patterns/1  "Switching Patterns"
  Constant4/1 -> Multiport Switch/4
  Constant1/1 -> Multiport Switch/2
  Constant7/1 -> Multiport Switch/7
  Constant3/1 -> Multiport Switch/3
  Constant6/1 -> Multiport Switch/5
  Constant5/1 -> Multiport Switch/6

== system BLDC_motor_control_v1/Controller ==
  error : Inport
  PID Controller1 : simulink/Continuous/PID Controller  Controller=PI  TimeDomain=Continuous-time  SampleTime=-1  IntegratorMethod=Forward Euler  FilterMethod=Forward Euler  Form=Parallel  UseFilter=on  ControllerParametersSource=internal  P=0.01  I=5  D=0  N=100  InitialConditionSource=internal  InitialConditionForIntegrator=0  InitialConditionForFilter=0  ExternalReset=none  LimitOutput=off  UpperSaturationLimit=inf  LowerSaturationLimit=-inf  LinearizeAsGain=on  AntiWindupMode=none  Kb=1  TrackingMode=off  Kt=1  PParamMin=[]  PParamMax=[]  IParamMin=[]  IParamMax=[]  DParamMin=[]  DParamMax=[]  NParamMin=[]  NParamMax=[]  KbParamMin=[]  KbParamMax=[]  KtParamMin=[]  KtParamMax=[]  POutMin=[]  POutMax=[]  IOutMin=[]  IOutMax=[]  DOutMin=[]  DOutMax=[]  NOutMin=[]  NOutMax=[]  KbOutMin=[]  KbOutMax=[]  KtOutMin=[]  KtOutMax=[]  IntegratorOutMin=[]  IntegratorOutMax=[]  FilterOutMin=[]  FilterOutMax=[]  SumOutMin=[]  SumOutMax=[]  SumI1OutMin=[]  SumI1OutMax=[]  SumI2OutMin=[]  SumI2OutMax=[]  SumI3OutMin=[]  SumI3OutMax=[]  SumDOutMin=[]  SumDOutMax=[]  SaturationOutMin=[]  SaturationOutMax=[]  IntegratorContinuousStateAttributes=''  IntegratorStateMustResolveToSignalObject=off  IntegratorRTWStateStorageClass=Auto  FilterContinuousStateAttributes=''  FilterStateMustResolveToSignalObject=off  FilterRTWStateStorageClass=Auto  DifferentiatorICPrevScaledInput=0  DifferentiatorOutMin=[]  DifferentiatorOutMax=[]  InitialConditionSetting=State (most efficient)  FilterDiffOutCoefMin=[]  FilterDiffOutCoefMax=[]  SumDenOutMin=[]  SumDenOutMax=[]  SumNumOutMin=[]  SumNumOutMax=[]  ReciprocalOutMin=[]  ReciprocalOutMax=[]  DivideOutMin=[]  DivideOutMax=[]  TunerSelectOption=Transfer Function Based (PID Tuner App)
  duty cycle : Outport
  wires:
  PID Controller1/1 -> duty cycle/1
  error/1 -> PID Controller1/1

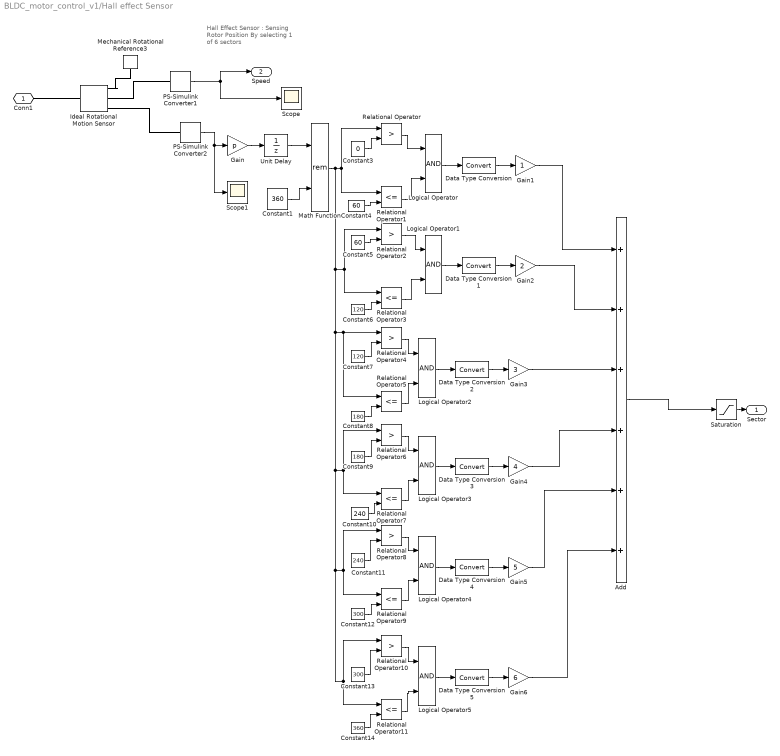
== system BLDC_motor_control_v1/Hall effect Sensor ==
  note: Hall Effect Sensor : Sensing Rotor Position By selecting 1 of 6 sectors
  Add : Sum  Inputs=++++++
  Constant1 : Constant  Value=360
  Constant10 : Constant  Value=240
  Constant11 : Constant  Value=240
  Constant12 : Constant  Value=300
  Constant13 : Constant  Value=300
  Constant14 : Constant  Value=360
  Constant3 : Constant  Value=0
  Constant4 : Constant  Value=60
  Constant5 : Constant  Value=60
  Constant6 : Constant  Value=120
  Constant7 : Constant  Value=120
  Constant8 : Constant  Value=180
  Constant9 : Constant  Value=180
  Data Type Conversion{,1..5} (6 alike) : DataTypeConversion
  Gain : Gain  Gain=p
  Gain1 : Gain
  Gain2 : Gain  Gain=2
  Gain3 : Gain  Gain=3
  Gain4 : Gain  Gain=4
  Gain5 : Gain  Gain=5
  Gain6 : Gain  Gain=6
  Ideal Rotational Motion Sensor : fl_lib/Mechanical/Mechanical Sensors/Ideal Rotational Motion Sensor  offset=0 deg
  Logical Operator{,1..5} (6 alike) : Logic  AllPortsSameDT=off  OutDataTypeStr=boolean
  Math Function : Math  Operator=rem  SaturateOnIntegerOverflow=on
  Mechanical Rotational Reference3 : fl_lib/Mechanical/Rotational Elements/Mechanical Rotational Reference
  PS-Simulink Converter1 : nesl_utility/PS-Simulink Converter  PhysicalDomain=network_engine_domain  SubClassName=ps_output  LeftPortType=input  RightPortType=output  PseudoPeriodic=off  Frequencies=[]  Unit=1  AffineConversion=off
  PS-Simulink Converter2 : nesl_utility/PS-Simulink Converter  PhysicalDomain=network_engine_domain  SubClassName=ps_output  LeftPortType=input  RightPortType=output  PseudoPeriodic=off  Frequencies=[]  Unit=1  AffineConversion=off
  Relational Operator{,2,4,6,8,10} (6 alike) : RelationalOperator  Operator=>  OutDataTypeStr=boolean  RndMeth=Simplest
  Relational Operator{1,3,5,7,9,11} (6 alike) : RelationalOperator  Operator=<=  OutDataTypeStr=boolean  RndMeth=Simplest
  Saturation : Saturate  UpperLimit=6  LowerLimit=1
  Scope : Scope
  Scope1 : Scope
  Unit Delay : UnitDelay  SampleTime=-1
  Conn1 : PMIOPort  Port=1  Side=Left
  Sector : Outport
  Speed : Outport  Port=2
  wires:
  PS-Simulink Converter1/1 -> Scope/1, Speed/1
  Constant4/1 -> Relational Operator1/2
  Constant3/1 -> Relational Operator/2
  Gain5/1 -> Add/5
  Logical Operator4/1 -> Data Type Conversion4/1
  Constant12/1 -> Relational Operator9/2
  Relational Operator8/1 -> Logical Operator4/1
  Data Type Conversion4/1 -> Gain5/1
  Constant11/1 -> Relational Operator8/2
  Relational Operator9/1 -> Logical Operator4/2
  Data Type Conversion/1 -> Gain1/1
  Relational Operator1/1 -> Logical Operator/2
  Constant10/1 -> Relational Operator7/2
  Relational Operator7/1 -> Logical Operator3/2
  Data Type Conversion3/1 -> Gain4/1
  Logical Operator3/1 -> Data Type Conversion3/1
  Constant9/1 -> Relational Operator6/2
  Gain4/1 -> Add/4
  Relational Operator6/1 -> Logical Operator3/1
  Unit Delay/1 -> Math Function/1
  Data Type Conversion1/1 -> Gain2/1
  Relational Operator3/1 -> Logical Operator1/2
  Gain2/1 -> Add/2
  Logical Operator1/1 -> Data Type Conversion1/1
  Constant6/1 -> Relational Operator3/2
  Relational Operator2/1 -> Logical Operator1/1
  Constant5/1 -> Relational Operator2/2
  Relational Operator11/1 -> Logical Operator5/2
  Math Function/1 -> Relational Operator/1, Relational Operator1/1, Relational Operator2/1, Relational Operator3/1, Relational Operator4/1, Relational Operator5/1, Relational Operator10/1, Relational Operator11/1, Relational Operator8/1, Relational Operator9/1, Relational Operator6/1, Relational Operator7/1
  Relational Operator10/1 -> Logical Operator5/1
  Logical Operator5/1 -> Data Type Conversion5/1
  Constant14/1 -> Relational Operator11/2
  Data Type Conversion5/1 -> Gain6/1
  Gain6/1 -> Add/6
  Constant13/1 -> Relational Operator10/2
  Relational Operator/1 -> Logical Operator/1
  Data Type Conversion2/1 -> Gain3/1
  Gain3/1 -> Add/3
  Logical Operator2/1 -> Data Type Conversion2/1
  Relational Operator4/1 -> Logical Operator2/1
  Relational Operator5/1 -> Logical Operator2/2
  Constant8/1 -> Relational Operator5/2
  Constant7/1 -> Relational Operator4/2
  Gain1/1 -> Add/1
  Saturation/1 -> Sector/1
  Logical Operator/1 -> Data Type Conversion/1
  Constant1/1 -> Math Function/2
  Gain/1 -> Unit Delay/1
  PS-Simulink Converter2/1 -> Scope1/1, Gain/1
  Add/1 -> Saturation/1
  connections:
  Ideal Rotational Motion Sensor/LConn1 -- Conn1/RConn1
  Ideal Rotational Motion Sensor/RConn3 -- PS-Simulink Converter2/LConn1
  Ideal Rotational Motion Sensor/RConn1 -- Mechanical Rotational Reference3/LConn1
  Ideal Rotational Motion Sensor/RConn2 -- PS-Simulink Converter1/LConn1

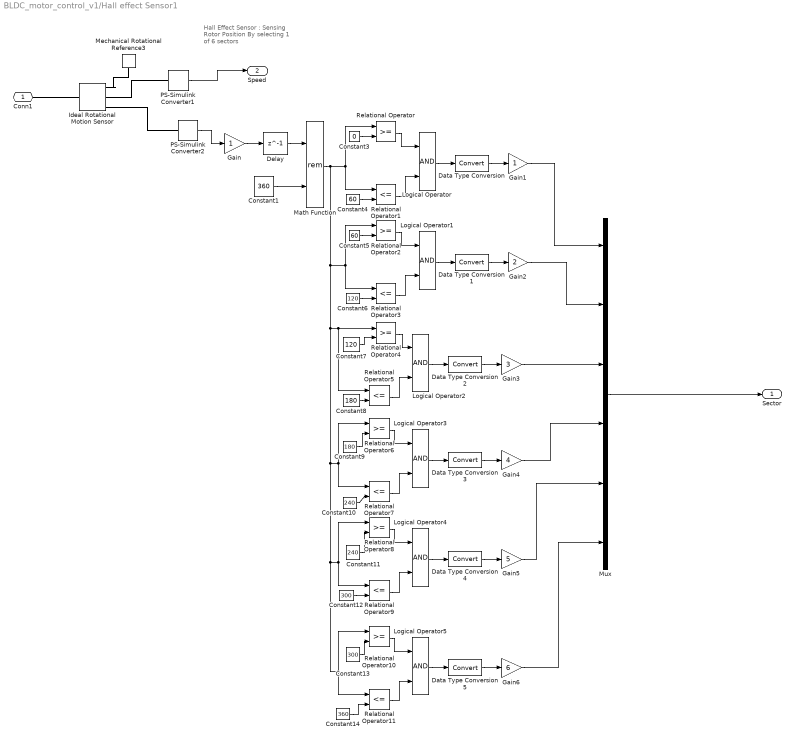
== system BLDC_motor_control_v1/Hall effect Sensor1 ==
  note: Hall Effect Sensor : Sensing Rotor Position By selecting 1 of 6 sectors
  Constant1 : Constant  Value=360
  Constant10 : Constant  Value=240
  Constant11 : Constant  Value=240
  Constant12 : Constant  Value=300
  Constant13 : Constant  Value=300
  Constant14 : Constant  Value=360
  Constant3 : Constant  Value=0
  Constant4 : Constant  Value=60
  Constant5 : Constant  Value=60
  Constant6 : Constant  Value=120
  Constant7 : Constant  Value=120
  Constant8 : Constant  Value=180
  Constant9 : Constant  Value=180
  Data Type Conversion{,1..5} (6 alike) : DataTypeConversion
  Delay : Delay  DelayLength=1
  Gain : Gain
  Gain1 : Gain
  Gain2 : Gain  Gain=2
  Gain3 : Gain  Gain=3
  Gain4 : Gain  Gain=4
  Gain5 : Gain  Gain=5
  Gain6 : Gain  Gain=6
  Ideal Rotational Motion Sensor : fl_lib/Mechanical/Mechanical Sensors/Ideal Rotational Motion Sensor  offset=0 rad
  Logical Operator{,1..5} (6 alike) : Logic  AllPortsSameDT=off  OutDataTypeStr=boolean
  Math Function : Math  Operator=rem  SaturateOnIntegerOverflow=on
  Mechanical Rotational Reference3 : fl_lib/Mechanical/Rotational Elements/Mechanical Rotational Reference
  Mux : Mux  Inputs=6
  PS-Simulink Converter1 : nesl_utility/PS-Simulink Converter  PhysicalDomain=network_engine_domain  SubClassName=ps_output  LeftPortType=input  RightPortType=output  PseudoPeriodic=off  Frequencies=[]  Unit=1  AffineConversion=off
  PS-Simulink Converter2 : nesl_utility/PS-Simulink Converter  PhysicalDomain=network_engine_domain  SubClassName=ps_output  LeftPortType=input  RightPortType=output  PseudoPeriodic=off  Frequencies=[]  Unit=1  AffineConversion=off
  Relational Operator{,2,4,6,8,10} (6 alike) : RelationalOperator  OutDataTypeStr=boolean  RndMeth=Simplest
  Relational Operator{1,3,5,7,9,11} (6 alike) : RelationalOperator  Operator=<=  OutDataTypeStr=boolean  RndMeth=Simplest
  Conn1 : PMIOPort  Port=1  Side=Left
  Sector : Outport
  Speed : Outport  Port=2
  wires:
  PS-Simulink Converter2/1 -> Gain/1
  Gain5/1 -> Mux/5
  Gain/1 -> Delay/1
  Gain6/1 -> Mux/6
  Relational Operator10/1 -> Logical Operator5/1
  Relational Operator6/1 -> Logical Operator3/1
  Data Type Conversion2/1 -> Gain3/1
  Logical Operator/1 -> Data Type Conversion/1
  Constant6/1 -> Relational Operator3/2
  Constant1/1 -> Math Function/2
  Relational Operator5/1 -> Logical Operator2/2
  Relational Operator/1 -> Logical Operator/1
  Relational Operator4/1 -> Logical Operator2/1
  Constant9/1 -> Relational Operator6/2
  Constant10/1 -> Relational Operator7/2
  Mux/1 -> Sector/1
  Constant3/1 -> Relational Operator/2
  Data Type Conversion1/1 -> Gain2/1
  Math Function/1 -> Relational Operator1/1, Relational Operator/1, Relational Operator3/1, Relational Operator2/1, Relational Operator5/1, Relational Operator4/1, Relational Operator11/1, Relational Operator10/1, Relational Operator9/1, Relational Operator8/1, Relational Operator7/1, Relational Operator6/1
  Gain2/1 -> Mux/2
  Constant8/1 -> Relational Operator5/2
  Relational Operator8/1 -> Logical Operator4/1
  Relational Operator2/1 -> Logical Operator1/1
  Gain4/1 -> Mux/4
  Logical Operator1/1 -> Data Type Conversion1/1
  Logical Operator2/1 -> Data Type Conversion2/1
  Gain3/1 -> Mux/3
  Delay/1 -> Math Function/1
  Gain1/1 -> Mux/1
  Logical Operator5/1 -> Data Type Conversion5/1
  Constant14/1 -> Relational Operator11/2
  Constant13/1 -> Relational Operator10/2
  Constant7/1 -> Relational Operator4/2
  Relational Operator11/1 -> Logical Operator5/2
  Data Type Conversion5/1 -> Gain6/1
  Data Type Conversion3/1 -> Gain4/1
  Relational Operator9/1 -> Logical Operator4/2
  Relational Operator7/1 -> Logical Operator3/2
  Relational Operator3/1 -> Logical Operator1/2
  Data Type Conversion/1 -> Gain1/1
  Logical Operator4/1 -> Data Type Conversion4/1
  Data Type Conversion4/1 -> Gain5/1
  Constant5/1 -> Relational Operator2/2
  Constant4/1 -> Relational Operator1/2
  Constant11/1 -> Relational Operator8/2
  PS-Simulink Converter1/1 -> Speed/1
  Logical Operator3/1 -> Data Type Conversion3/1
  Relational Operator1/1 -> Logical Operator/2
  Constant12/1 -> Relational Operator9/2
  connections:
  Ideal Rotational Motion Sensor/RConn3 -- PS-Simulink Converter2/LConn1
  Ideal Rotational Motion Sensor/RConn2 -- PS-Simulink Converter1/LConn1
  Ideal Rotational Motion Sensor/LConn1 -- Conn1/RConn1
  Ideal Rotational Motion Sensor/RConn1 -- Mechanical Rotational Reference3/LConn1
